simulink model "CAT797_lateral_dynamics_differential_flatness_control_control_loop_carla_bridge"  (R2025a)
settings: Solver=FixedStepAuto  StartTime=0.0  StopTime=150  FixedStep=0.01  RelTol=1e-3
PreLoadFcn:
  | clc; clear;
  | py_folder = 'G:\Control_Research\Autonomy_Mining_Dump_Truck\src\sim';
  | if count(py.sys.path, py_folder) == 0
  |     insert(py.sys.path, int32(0), py_folder);
  | end
  | py.importlib.invalidate_caches();
  | % NOTE: do NOT call import_module here — setupImpl loads the exact file
  | addpath("G:\Control_Research\Autonomy_Mining_Dump_Truck\src\plant_model\lib")
undefined symbols (not defined in the file or in its folder): Cf, Cr, Iz, k0, k1, ki, ky, Lf, Lr
libraries: slpidlib x1
settings Model: DataDictionary=CAT_797F.sldd  Creator=marti343  LastModifiedBy=marti343
settings OptimizationCC: EnableMemcpy=off
settings HardwareCC: ProdBitPerChar=16.0  ProdBitPerInt=16.0  ProdBitPerPointer=32.0  ProdBitPerSizeT=32.0  ProdBitPerPtrDiffT=32.0  ProdLargestAtomicInteger=Integer  ProdLargestAtomicFloat=None  ProdWordSize=16.0  ProdHWDeviceType=Texas Instruments->C2000
settings RTWCC: GenerateReport=on  LaunchReport=on
settings CodeAppCC: ForceParamTrailComments=on  StateflowObjectComments=on  MATLABSourceComments=on

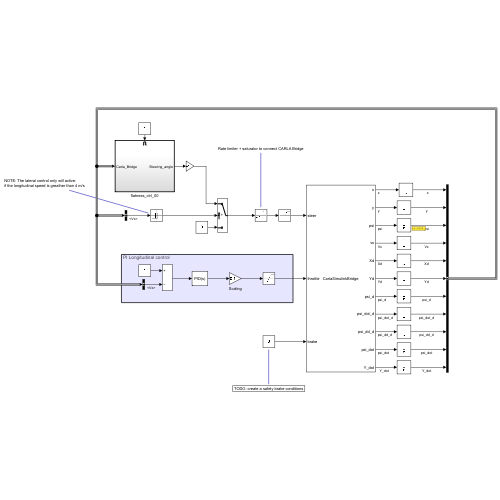
[thumbnail: Simulink's stored preview of the top-level diagram]
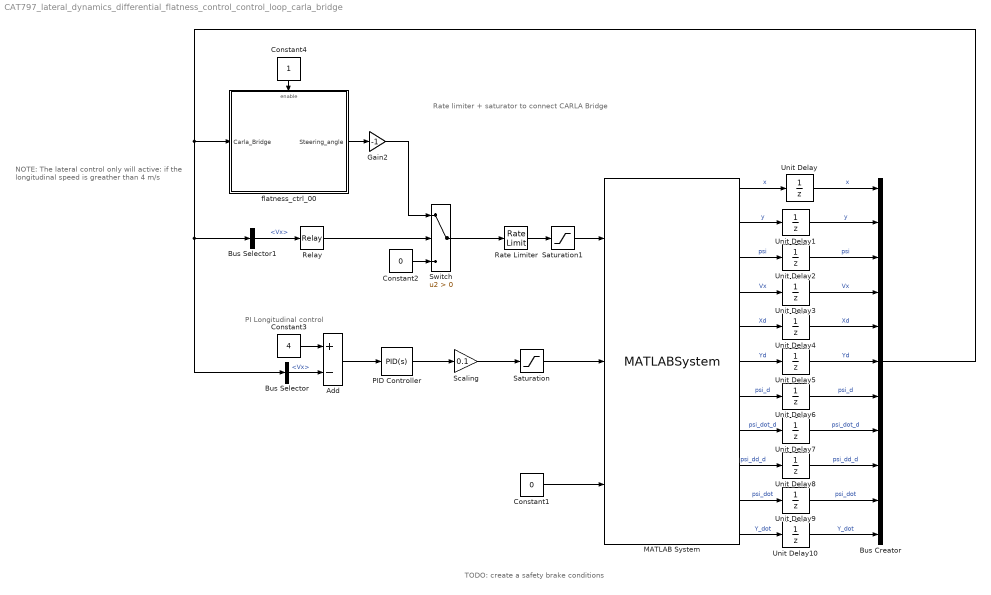
== system CAT797_lateral_dynamics_differential_flatness_control_control_loop_carla_bridge ==
  note: TODO: create a safety brake conditions
  note: Rate limiter + saturator to connect CARLA Bridge
  note: NOTE: The lateral control only will active:
      | if the longitudinal speed is greather than 4 m/s
  note: PI Longitudinal control
  Add : Sum  Inputs=+-
  Bus Creator : BusCreator  Inputs=11
  Bus Selector : BusSelector  OutputSignals=Vx
  Bus Selector1 : BusSelector  OutputSignals=Vx
  Constant1 : Constant  Value=0  SampleTime=-1
  Constant2 : Constant  Value=0
  Constant3 : Constant  Value=4
  Constant4 : Constant
  Gain2 : Gain  Gain=-1
  MATLAB System : MATLABSystem  System=CarlaSimulinkBridge  PythonFolder=G:\Control_Research\Autonomy_Mining_Dump_Truck\src\plant_model  SimulateUsing=Interpreted execution
      mask Type: CarlaSimulinkBridge
  PID Controller : slpidlib/PID Controller  Controller=PID  Form=Parallel  TimeDomain=Continuous-time  UseExternalTs=off  SampleTime=-1  IntegratorMethod=Forward Euler  FilterMethod=Forward Euler  ControllerParametersSource=internal  P=0.3  I=0.5  UseKiTs=off  D=0  UseExternalDerivativeSource=off  N=100  UseFilter=on  TunerSelectOption=Transfer Function Based (PID Tuner App)  InitialConditionSource=internal  InitialConditionForIntegrator=0  InitialConditionForFilter=0  DifferentiatorICPrevScaledInput=0  ExternalReset=none  TrackingMode=off  Kt=1  LimitOutput=off  SatLimitsSource=internal  UpperSaturationLimit=inf  LowerSaturationLimit=-inf  LinearizeAsGain=on  AntiWindupMode=none  Kb=1  LimitIntegrator=off  UpperIntegratorSaturationLimit=inf  LowerIntegratorSaturationLimit=-inf  POutMin=[]  POutMax=[]  IOutMin=[]  IOutMax=[]  DOutMin=[]  DOutMax=[]  NOutMin=[]  NOutMax=[]  SumOutMin=[]  SumOutMax=[]  SaturationOutMin=[]  SaturationOutMax=[]  PParamMin=[]  PParamMax=[]  IParamMin=[]  IParamMax=[]  DParamMin=[]  DParamMax=[]  NParamMin=[]  NParamMax=[]  KbParamMin=[]  KbParamMax=[]  KtParamMin=[]  KtParamMax=[]  KbOutMin=[]  KbOutMax=[]  KtOutMin=[]  KtOutMax=[]  IntegratorOutMin=[]  IntegratorOutMax=[]  FilterOutMin=[]  FilterOutMax=[]  SumI1OutMin=[]  SumI1OutMax=[]  SumI2OutMin=[]  SumI2OutMax=[]  SumI3OutMin=[]  SumI3OutMax=[]  SumI4OutMin=[]  SumI4OutMax=[]  SumDOutMin=[]  SumDOutMax=[]  DifferentiatorOutMin=[]  DifferentiatorOutMax=[]  FilterDiffOutCoefMin=[]  FilterDiffOutCoefMax=[]  ReciprocalOutMin=[]  ReciprocalOutMax=[]  SumDenOutMin=[]  SumDenOutMax=[]  SumNumOutMin=[]  SumNumOutMax=[]  DivideOutMin=[]  DivideOutMax=[]  UdiffTsProdOutMin=[]  UdiffTsProdOutMax=[]  NTsProdOutMin=[]  NTsProdOutMax=[]  UintegralTsProdOutMin=[]  UintegralTsProdOutMax=[]  UngainTsProdOutMin=[]  UngainTsProdOutMax=[]  ClampingZeroOutDataTypeStr=Inherit: Inherit via back propagation  ClampingZeroOutMin=[]  ClampingZeroOutMax=[]  FilterDenConstantOutDataTypeStr=Inherit: Inherit via back propagation  FilterDenConstantOutMin=[]  FilterDenConstantOutMax=[]  PCopyOutDataTypeStr=Inherit: Inherit via back propagation  PCopyOutMin=[]  PCopyOutMax=[]  NCopyOutDataTypeStr=Inherit: Inherit via back propagation  NCopyOutMin=[]  NCopyOutMax=[]  IntegratorContinuousStateAttributes=''  IntegratorStateMustResolveToSignalObject=off  IntegratorRTWStateStorageClass=Auto  FilterContinuousStateAttributes=''  FilterStateMustResolveToSignalObject=off  FilterRTWStateStorageClass=Auto  ParallelPVariant=InternalParameters  IdealPVariant=Disabled  IVariant=InternalParameters  DVariant=InternalParameters  IntegratorVariant=Continuous  SatVariant=Disabled  AWVariant=Passthrough  PCopyVariant=Disabled  TRVariant=Disabled  FdbkBlocksVariant=Forward  IdealPFdbkVariant=Disabled  SatFdbkVariant=Disabled  DerivativeFilterVariant=ContFilter  NVariant=InternalParameters  NCopyVariant=Disabled  FilterICVariant=InternalICsFilter  IntegratorICVariant=InternalICs  ExternalResetVariant=Disabled  TRSumVariant=Passthrough  SumFdbkVariant=Disabled  SumVariant=Sum_PID  TsampFilterVariant=InternalTs  TsampNgainVariant=Passthrough  TsampIntegralVariant=Disabled_SignalSpec  ExternalSaturationOutDataTypeStr=Inherit: Same as second input  DerivativeSourceVariant=ErrorSignal  PreIntVariant=InternalPreInt
  Rate Limiter : RateLimiter  RisingSlewLimit=3  FallingSlewLimit=-3  SampleTimeMode=inherited
  Relay : Relay  OnSwitchValue=4  OffSwitchValue=0.5
  Saturation : Saturate  UpperLimit=1  LowerLimit=0
  Saturation1 : Saturate  UpperLimit=1  LowerLimit=-1
  Scaling : Gain  Gain=0.1
  Switch : Switch  Criteria=u2 > Threshold  SaturateOnIntegerOverflow=off  InputSameDT=off
  Unit Delay{,1..10} (11 alike) : UnitDelay  SampleTime=0.01  HasFrameUpgradeWarning=on
  flatness_ctrl_00 : Subsystem
  wires:
  Constant1/1 -> MATLAB System/3
  PID Controller/1 -> Scaling/1
  MATLAB System/4 -> Unit Delay3/1  "Vx"
  MATLAB System/5 -> Unit Delay4/1  "Xd"
  MATLAB System/6 -> Unit Delay5/1  "Yd"
  MATLAB System/7 -> Unit Delay6/1  "psi_d"
  MATLAB System/8 -> Unit Delay7/1  "psi_dot_d"
  MATLAB System/9 -> Unit Delay8/1  "psi_dd_d"
  MATLAB System/1 -> Unit Delay/1  "x"
  MATLAB System/2 -> Unit Delay1/1  "y"
  MATLAB System/3 -> Unit Delay2/1  "psi"
  Bus Creator/1 -> Bus Selector/1, Bus Selector1/1, flatness_ctrl_00/1(Carla_Bridge)
  MATLAB System/10 -> Unit Delay9/1  "psi_dot"
  MATLAB System/11 -> Unit Delay10/1  "Y_dot"
  Unit Delay/1 -> Bus Creator/1  "x"
  Unit Delay1/1 -> Bus Creator/2  "y"
  Unit Delay2/1 -> Bus Creator/3  "psi"
  Unit Delay3/1 -> Bus Creator/4  "Vx"
  Unit Delay4/1 -> Bus Creator/5  "Xd"
  Unit Delay5/1 -> Bus Creator/6  "Yd"
  Unit Delay6/1 -> Bus Creator/7  "psi_d"
  Unit Delay7/1 -> Bus Creator/8  "psi_dot_d"
  Unit Delay8/1 -> Bus Creator/9  "psi_dd_d"
  Unit Delay9/1 -> Bus Creator/10  "psi_dot"
  Unit Delay10/1 -> Bus Creator/11  "Y_dot"
  Saturation/1 -> MATLAB System/2
  Constant3/1 -> Add/1
  Bus Selector/1 -> Add/2  "<Vx>"
  Add/1 -> PID Controller/1
  Saturation1/1 -> MATLAB System/1
  Scaling/1 -> Saturation/1
  Bus Selector1/1 -> Relay/1  "<Vx>"
  Relay/1 -> Switch/2
  Constant2/1 -> Switch/3
  Constant4/1 -> flatness_ctrl_00/Enable
  Rate Limiter/1 -> Saturation1/1
  flatness_ctrl_00/1(Steering_angle) -> Gain2/1
  Switch/1 -> Rate Limiter/1
  Gain2/1 -> Switch/1

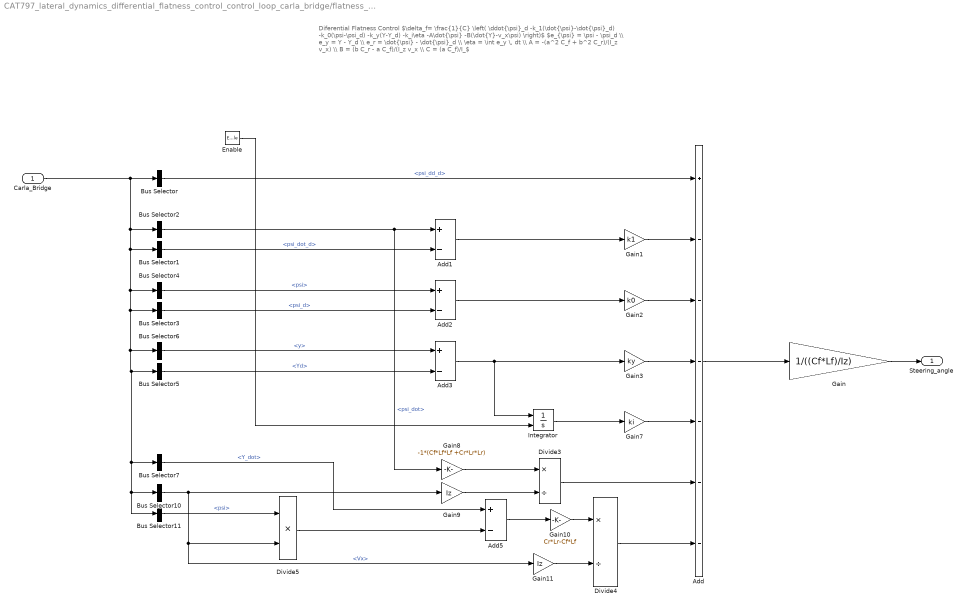
== system CAT797_lateral_dynamics_differential_flatness_control_control_loop_carla_bridge/flatness_ctrl_00 ==
  note: Diferential Flatness Control
      |
      | $\delta_f= \frac{1}{C} \left( \ddot{\psi}_d -k_1(\dot{\psi}-\dot{\psi}_d) -k_0(\psi-\psi_d) -k_y(Y-Y_d) -k_i\eta -A\dot{\psi} -B(\dot{Y}-v_x\psi) \right)$
      |
      | $e_{\psi} = \psi - \psi_d \\ e_y = Y - Y_d \\ e_r = \dot{\psi} - \dot{\psi}_d \\ \eta = \int e_y \, dt \\ A = -(a^2 C_f + b^2 C_r)/(I_z v_x) \\ B = (b C_r - a C_f)/(I_z v_x \\ C = (a C_f)/I_$
  Carla_Bridge : Inport
  Enable : EnablePort  ShowOutputPort=on
  Add : Sum  Inputs=+------
  Add{1..3,5} (4 alike) : Sum  Inputs=+-
  Bus Selector : BusSelector  OutputSignals=psi_dd_d
  Bus Selector1 : BusSelector  OutputSignals=psi_dot_d
  Bus Selector10 : BusSelector  OutputSignals=Vx
  Bus Selector11 : BusSelector  OutputSignals=psi
  Bus Selector2 : BusSelector  OutputSignals=psi_dot
  Bus Selector3 : BusSelector  OutputSignals=psi_d
  Bus Selector4 : BusSelector  OutputSignals=psi
  Bus Selector5 : BusSelector  OutputSignals=Yd
  Bus Selector6 : BusSelector  OutputSignals=y
  Bus Selector7 : BusSelector  OutputSignals=Y_dot
  Divide3 : Product  Inputs=*/
  Divide4 : Product  Inputs=*/
  Divide5 : Product  Inputs=**
  Gain : Gain  Gain=1/((Cf*Lf)/Iz)
  Gain1 : Gain  Gain=k1
  Gain10 : Gain  Gain=Cr*Lr-Cf*Lf
  Gain11 : Gain  Gain=Iz
  Gain2 : Gain  Gain=k0
  Gain3 : Gain  Gain=ky
  Gain7 : Gain  Gain=ki
  Gain8 : Gain  Gain=-1*(Cf*Lf*Lf +Cr*Lr*Lr)
  Gain9 : Gain  Gain=Iz
  Integrator : Integrator  InitialConditionSource=external
  Steering_angle : Outport
  wires:
  Add/1 -> Gain/1
  Gain2/1 -> Add/3
  Add3/1 -> Integrator/1, Gain3/1
  Carla_Bridge/1 -> Bus Selector4/1, Bus Selector7/1, Bus Selector11/1, Bus Selector10/1, Bus Selector5/1, Bus Selector6/1, Bus Selector3/1, Bus Selector1/1, Bus Selector2/1, Bus Selector/1
  Bus Selector4/1 -> Add2/1  "<psi>"
  Bus Selector1/1 -> Add1/2  "<psi_dot_d>"
  Bus Selector5/1 -> Add3/2  "<Yd>"
  Gain1/1 -> Add/2
  Add2/1 -> Gain2/1
  Gain/1 -> Steering_angle/1
  Gain3/1 -> Add/4
  Bus Selector6/1 -> Add3/1  "<y>"
  Add1/1 -> Gain1/1
  Bus Selector3/1 -> Add2/2  "<psi_d>"
  Integrator/1 -> Gain7/1
  Bus Selector/1 -> Add/1  "<psi_dd_d>"
  Bus Selector2/1 -> Gain8/1, Add1/1  "<psi_dot>"
  Gain7/1 -> Add/5
  Gain9/1 -> Divide3/2
  Gain8/1 -> Divide3/1
  Divide3/1 -> Add/6
  Bus Selector10/1 -> Gain9/1, Gain11/1, Divide5/2  "<Vx>"
  Gain10/1 -> Divide4/1
  Gain11/1 -> Divide4/2
  Add5/1 -> Gain10/1
  Divide5/1 -> Add5/2
  Divide4/1 -> Add/7
  Bus Selector11/1 -> Divide5/1  "<psi>"
  Bus Selector7/1 -> Add5/1  "<Y_dot>"
  Enable/1 -> Integrator/2
